simulink model "heat_transfer_for_TEM"  (R2019a)
settings: Solver=VariableStepAuto  StartTime=0.0  StopTime=200  RelTol=1e-3
libraries: Lib_Solve_SSNRSolverJC_TMATS x2
settings Model: Creator=student  LastModifiedBy=student

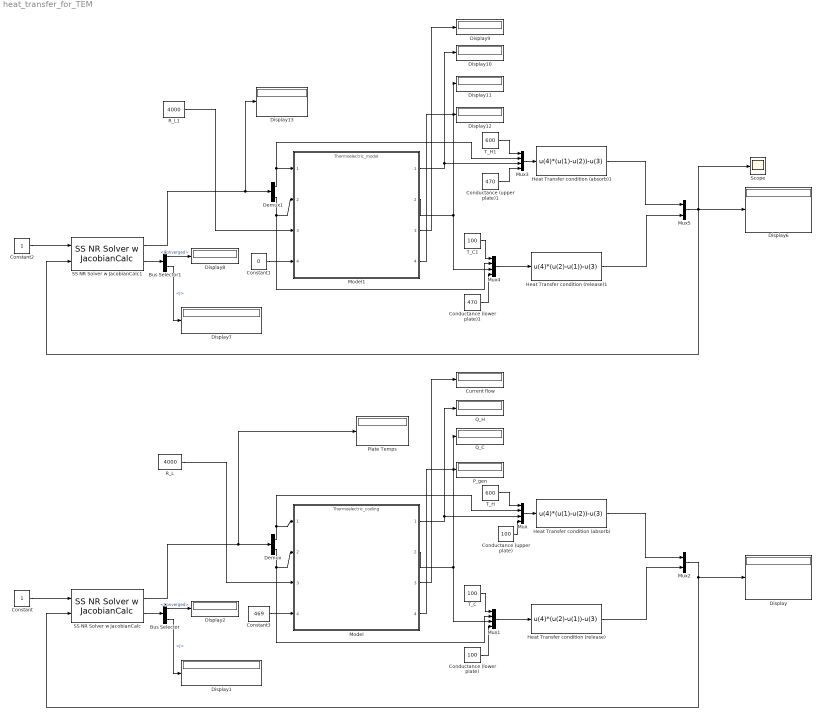
== system heat_transfer_for_TEM ==
  Bus Selector : BusSelector  OutputSignals=Converged,J
  Bus Selector1 : BusSelector  OutputSignals=Converged,J
  Conductance (lower plate) : Constant  Value=100
  Conductance (lower plate)1 : Constant  Value=470
  Conductance (upper plate) : Constant  Value=100
  Conductance (upper plate)1 : Constant  Value=470
  Constant : Constant
  Constant1 : Constant  Value=0
  Constant2 : Constant
  Constant3 : Constant  Value=469
  Current flow : Display
  Demux : Demux  Outputs=2
  Demux1 : Demux  Outputs=2
  Display{,1..2,6..13} (11 alike) : Display
  Heat Transfer condition (absorb) : Fcn  Expr=u(4)*(u(1)-u(2))-u(3)
  Heat Transfer condition (absorb)1 : Fcn  Expr=u(4)*(u(1)-u(2))-u(3)
  Heat Transfer condition (release) : Fcn  Expr=u(4)*(u(2)-u(1))-u(3)
  Heat Transfer condition (release)1 : Fcn  Expr=u(4)*(u(2)-u(1))-u(3)
  Model : ModelReference  ModelNameDialog=Thermoelectric_cooling.slx  SimulationMode=Normal  ModelReferenceVersion=1.18
  Model1 : ModelReference  ModelNameDialog=Thermoelectric_model.slx  SimulationMode=Normal  ModelReferenceVersion=1.18
  Mux{,1,3..4} (4 alike) : Mux
  Mux2 : Mux  Inputs=2
  Mux5 : Mux  Inputs=2
  P_gen : Display
  Plate Temps : Display
  Q_C : Display
  Q_H : Display
  R_L : Constant  Value=4000
  R_L1 : Constant  Value=4000
  SS NR Solver w JacobianCalc : Lib_Solve_SSNRSolverJC_TMATS/SS NR Solver w JacobianCalc  SJac_Per_M=0.05*[1 1]  SNR_IC_M=[1 700]  SNR_DX_M=5  SNR_Mx_M=100000  SNR_Mn_M=0.00001  SJacobianAttempts_M=20  Cond_Limits_M=0.0001
  SS NR Solver w JacobianCalc1 : Lib_Solve_SSNRSolverJC_TMATS/SS NR Solver w JacobianCalc  SJac_Per_M=0.05*[1 1]  SNR_IC_M=[300 300]  SNR_DX_M=20  SNR_Mx_M=100000  SNR_Mn_M=0.0001  SJacobianAttempts_M=5  Cond_Limits_M=.0001
  Scope : Scope
  T_C : Constant  Value=100
  T_C1 : Constant  Value=100
  T_H : Constant  Value=600
  T_H1 : Constant  Value=600
  wires:
  Mux1/1 -> Heat Transfer condition (release)/1
  Mux/1 -> Heat Transfer condition (absorb)/1
  Demux/1 -> Mux/2, Model/1
  Demux/2 -> Mux1/2, Model/2
  Heat Transfer condition (absorb)/1 -> Mux2/1
  Heat Transfer condition (release)/1 -> Mux2/2
  Mux2/1 -> SS NR Solver w JacobianCalc/2, Display/1
  Constant/1 -> SS NR Solver w JacobianCalc/1
  SS NR Solver w JacobianCalc/2 -> Bus Selector/1
  Bus Selector/2 -> Display1/1  "<J>"
  Bus Selector/1 -> Display2/1  "<Converged>"
  Model/2 -> Mux1/3, Q_C/1
  Model/1 -> Q_H/1, Mux/3
  T_C/1 -> Mux1/1
  T_H/1 -> Mux/1
  Conductance (upper plate)/1 -> Mux/4
  Conductance (lower plate)/1 -> Mux1/4
  Model/3 -> Current flow/1
  R_L/1 -> Model/3
  Mux4/1 -> Heat Transfer condition (release)1/1
  Demux1/1 -> Mux3/2, Model1/1
  Model1/3 -> Display9/1
  Heat Transfer condition (release)1/1 -> Mux5/2
  Demux1/2 -> Mux4/2, Model1/2
  Heat Transfer condition (absorb)1/1 -> Mux5/1
  Mux5/1 -> SS NR Solver w JacobianCalc1/2, Display6/1, Scope/1
  Constant2/1 -> SS NR Solver w JacobianCalc1/1
  Bus Selector1/1 -> Display8/1  "<Converged>"
  Bus Selector1/2 -> Display7/1  "<J>"
  Model1/2 -> Mux4/3, Display11/1
  SS NR Solver w JacobianCalc1/2 -> Bus Selector1/1
  Mux3/1 -> Heat Transfer condition (absorb)1/1
  T_C1/1 -> Mux4/1
  Conductance (lower plate)1/1 -> Mux4/4
  Model1/1 -> Display10/1, Mux3/3
  SS NR Solver w JacobianCalc1/1 -> Display13/1, Demux1/1
  T_H1/1 -> Mux3/1
  Conductance (upper plate)1/1 -> Mux3/4
  R_L1/1 -> Model1/3
  Model1/4 -> Display12/1
  Model/4 -> P_gen/1
  SS NR Solver w JacobianCalc/1 -> Plate Temps/1, Demux/1
  Constant1/1 -> Model1/4
  Constant3/1 -> Model/4
